simulink model "Longitudinal_Simulink_MaskedParameter"  (Simulink 7.1)
settings: Solver=ode45  StartTime=0.0  StopTime=1.0  RelTol=1e-3
settings Model: Creator=Meisel  LastModifiedBy=Meisel

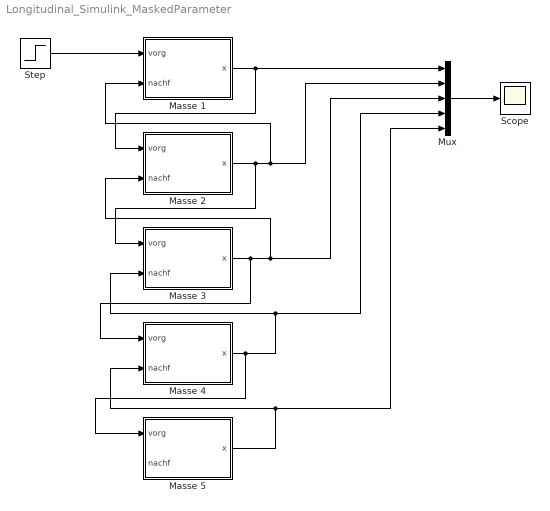
== system Longitudinal_Simulink_MaskedParameter ==
  Masse 1 : Subsystem  mask{Init_Pos=0}
      mask prompts: Init_Pos "Startposition"
  Masse 2 : Subsystem  mask{Init_Pos=0}
      mask prompts: Init_Pos "Startposition"
  Masse 3 : Subsystem  mask{Init_Pos=0}
      mask prompts: Init_Pos "Startposition"
  Masse 4 : Subsystem  mask{Init_Pos=0}
      mask prompts: Init_Pos "Startposition"
  Masse 5 : Subsystem  mask{Init_Pos=0}
      mask prompts: Init_Pos "Startposition"
  Mux : Mux  Inputs=5
  Scope : Scope
      settings: TimeRange=1  YMin=0  YMax=6
  Step : Step  Time=0.1  After=0.5  SampleTime=0
  wires:
  Masse 1/1(x) -> Mux/1, Masse 2/1(vorg)
  Step/1 -> Masse 1/1(vorg)
  Mux/1 -> Scope/1
  Masse 2/1(x) -> Masse 3/1(vorg), Masse 1/2(nachf), Mux/2
  Masse 3/1(x) -> Masse 4/1(vorg), Masse 2/2(nachf), Mux/3
  Masse 4/1(x) -> Masse 5/1(vorg), Masse 3/2(nachf), Mux/4
  Masse 5/1(x) -> Masse 4/2(nachf), Mux/5

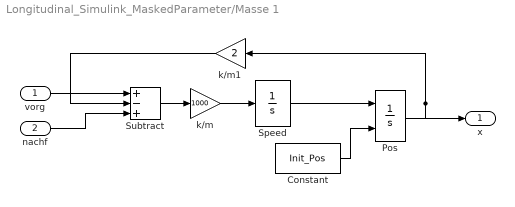
== system Longitudinal_Simulink_MaskedParameter/Masse 1 ==
  vorg : Inport  OutDataType=sfix(16)  OutScaling=2^0
  nachf : Inport  Port=2  OutDataType=sfix(16)  OutScaling=2^0
  Constant : Constant  Value=Init_Pos  OutDataType=sfix(16)  OutScaling=2^0
  Pos : Integrator  InitialConditionSource=external  InitialCondition=1
  Speed : Integrator
  Subtract : Sum  Inputs=+-+  OutDataType=sfix(16)  OutScaling=2^-10
  k/m : Gain  Gain=1000  ParameterDataType=sfix(16)  ParameterScaling=2^0  OutDataType=sfix(16)  OutScaling=2^0
  k/m1 : Gain  Orientation=left  Gain=2  ParameterDataType=sfix(16)  ParameterScaling=2^0  OutDataType=sfix(16)  OutScaling=2^0
  x : Outport  OutDataType=sfix(16)  OutScaling=2^0
  wires:
  Speed/1 -> Pos/1
  Subtract/1 -> k/m/1
  k/m/1 -> Speed/1
  Pos/1 -> x/1, k/m1/1
  nachf/1 -> Subtract/3
  vorg/1 -> Subtract/1
  k/m1/1 -> Subtract/2
  Constant/1 -> Pos/2

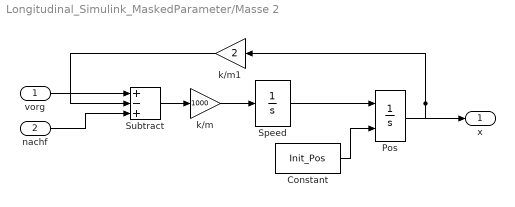
== system Longitudinal_Simulink_MaskedParameter/Masse 2 ==
  vorg : Inport  OutDataType=sfix(16)  OutScaling=2^0
  nachf : Inport  Port=2  OutDataType=sfix(16)  OutScaling=2^0
  Constant : Constant  Value=Init_Pos  OutDataType=sfix(16)  OutScaling=2^0
  Pos : Integrator  InitialConditionSource=external  InitialCondition=1
  Speed : Integrator
  Subtract : Sum  Inputs=+-+  OutDataType=sfix(16)  OutScaling=2^-10
  k/m : Gain  Gain=1000  ParameterDataType=sfix(16)  ParameterScaling=2^0  OutDataType=sfix(16)  OutScaling=2^0
  k/m1 : Gain  Orientation=left  Gain=2  ParameterDataType=sfix(16)  ParameterScaling=2^0  OutDataType=sfix(16)  OutScaling=2^0
  x : Outport  OutDataType=sfix(16)  OutScaling=2^0
  wires:
  Speed/1 -> Pos/1
  Subtract/1 -> k/m/1
  k/m/1 -> Speed/1
  Pos/1 -> x/1, k/m1/1
  nachf/1 -> Subtract/3
  vorg/1 -> Subtract/1
  k/m1/1 -> Subtract/2
  Constant/1 -> Pos/2

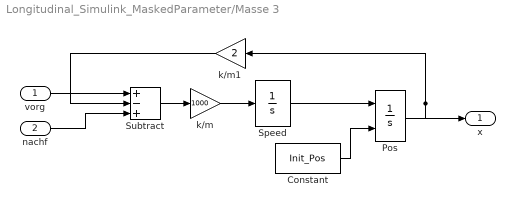
== system Longitudinal_Simulink_MaskedParameter/Masse 3 ==
  vorg : Inport  OutDataType=sfix(16)  OutScaling=2^0
  nachf : Inport  Port=2  OutDataType=sfix(16)  OutScaling=2^0
  Constant : Constant  Value=Init_Pos  OutDataType=sfix(16)  OutScaling=2^0
  Pos : Integrator  InitialConditionSource=external  InitialCondition=1
  Speed : Integrator
  Subtract : Sum  Inputs=+-+  OutDataType=sfix(16)  OutScaling=2^-10
  k/m : Gain  Gain=1000  ParameterDataType=sfix(16)  ParameterScaling=2^0  OutDataType=sfix(16)  OutScaling=2^0
  k/m1 : Gain  Orientation=left  Gain=2  ParameterDataType=sfix(16)  ParameterScaling=2^0  OutDataType=sfix(16)  OutScaling=2^0
  x : Outport  OutDataType=sfix(16)  OutScaling=2^0
  wires:
  Speed/1 -> Pos/1
  Subtract/1 -> k/m/1
  k/m/1 -> Speed/1
  Pos/1 -> x/1, k/m1/1
  nachf/1 -> Subtract/3
  vorg/1 -> Subtract/1
  k/m1/1 -> Subtract/2
  Constant/1 -> Pos/2

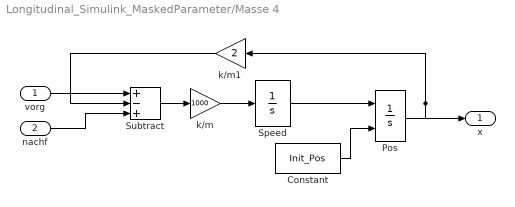
== system Longitudinal_Simulink_MaskedParameter/Masse 4 ==
  vorg : Inport  OutDataType=sfix(16)  OutScaling=2^0
  nachf : Inport  Port=2  OutDataType=sfix(16)  OutScaling=2^0
  Constant : Constant  Value=Init_Pos  OutDataType=sfix(16)  OutScaling=2^0
  Pos : Integrator  InitialConditionSource=external  InitialCondition=1
  Speed : Integrator
  Subtract : Sum  Inputs=+-+  OutDataType=sfix(16)  OutScaling=2^-10
  k/m : Gain  Gain=1000  ParameterDataType=sfix(16)  ParameterScaling=2^0  OutDataType=sfix(16)  OutScaling=2^0
  k/m1 : Gain  Orientation=left  Gain=2  ParameterDataType=sfix(16)  ParameterScaling=2^0  OutDataType=sfix(16)  OutScaling=2^0
  x : Outport  OutDataType=sfix(16)  OutScaling=2^0
  wires:
  Speed/1 -> Pos/1
  Subtract/1 -> k/m/1
  k/m/1 -> Speed/1
  Pos/1 -> x/1, k/m1/1
  nachf/1 -> Subtract/3
  vorg/1 -> Subtract/1
  k/m1/1 -> Subtract/2
  Constant/1 -> Pos/2

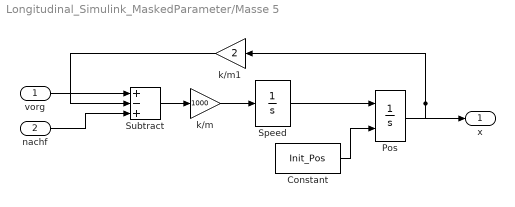
== system Longitudinal_Simulink_MaskedParameter/Masse 5 ==
  vorg : Inport  OutDataType=sfix(16)  OutScaling=2^0
  nachf : Inport  Port=2  OutDataType=sfix(16)  OutScaling=2^0
  Constant : Constant  Value=Init_Pos  OutDataType=sfix(16)  OutScaling=2^0
  Pos : Integrator  InitialConditionSource=external  InitialCondition=1
  Speed : Integrator
  Subtract : Sum  Inputs=+-+  OutDataType=sfix(16)  OutScaling=2^-10
  k/m : Gain  Gain=1000  ParameterDataType=sfix(16)  ParameterScaling=2^0  OutDataType=sfix(16)  OutScaling=2^0
  k/m1 : Gain  Orientation=left  Gain=2  ParameterDataType=sfix(16)  ParameterScaling=2^0  OutDataType=sfix(16)  OutScaling=2^0
  x : Outport  OutDataType=sfix(16)  OutScaling=2^0
  wires:
  Speed/1 -> Pos/1
  Subtract/1 -> k/m/1
  k/m/1 -> Speed/1
  Pos/1 -> x/1, k/m1/1
  nachf/1 -> Subtract/3
  vorg/1 -> Subtract/1
  k/m1/1 -> Subtract/2
  Constant/1 -> Pos/2
